simulink model "simulink_MPC"  (R2015a)
settings: Solver=ode45  StartTime=0.0  StopTime=0.015  RelTol=1e-3
values from neighbouring files (symbols this model uses):
  Ts = 1    [initialization_mpc.m]    (also in mpc_model.m = 0.01; mpc_model_working.m = 0.2; mpc_no_linear_model2.m = 0.005)
undefined symbols (not defined in the file or in its folder): alpha, Ao, Bo, Co, Do
settings Model: Creator=estudiante  LastModifiedBy=berme_000

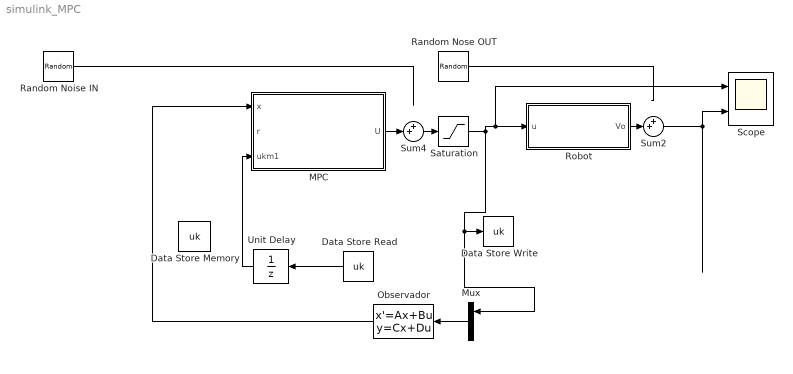
== system simulink_MPC ==
  Data Store Memory : DataStoreMemory  DataStoreName=uk  ReadBeforeWriteMsg=warning  WriteAfterWriteMsg=warning  WriteAfterReadMsg=warning
  Data Store Read : DataStoreRead  DataStoreName=uk
  Data Store Write : DataStoreWrite  DialogController=Simulink.DDGSource  DataStoreName=uk
  MPC : Subsystem
  Mux : Mux  Inputs=2
  Observador : StateSpace  A=Ao  B=Bo  C=Co  D=Do  X0=0
  Random Noise IN : RandomNumber  Variance=.0001  SampleTime=0.0001
  Random Nose OUT : RandomNumber  Variance=0.001  SampleTime=0.0001
  "Robot " : Subsystem
  Saturation : Saturate  UpperLimit=1-alpha  LowerLimit=0.5-alpha
  Scope : Scope  NumInputPorts=2
      settings: TimeRange=0.015  YMin=0.461212~-0.06  YMax=0.50976~0.07
  Sum2 : Sum  Inputs=++|
  Sum4 : Sum  Inputs=++|
  Unit Delay : UnitDelay  SampleTime=-1
  wires:
  Unit Delay/1 -> MPC/3(ukm1)
  Data Store Read/1 -> Unit Delay/1
  Observador/1 -> MPC/1(x)
  Mux/1 -> Observador/1
  Sum2/1 -> Scope/2
  Saturation/1 -> Mux/1, Data Store Write/1, "Robot "/1(u), Scope/1
  MPC/1(U) -> Sum4/2
  Random Noise IN/1 -> ?
  Sum4/1 -> Saturation/1
  "Robot "/1(Vo) -> Sum2/2
  Random Nose OUT/1 -> ?

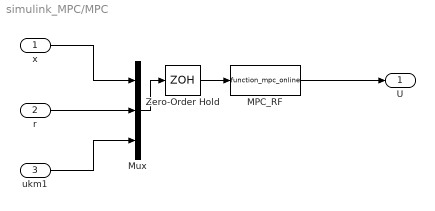
== system simulink_MPC/MPC ==
  x : Inport  PortDimensions=4
  r : Inport  Port=2
  ukm1 : Inport  Port=3
  MPC_RF : MATLABFcn  MATLABFcn=function_mpc_online
  Mux : Mux  Inputs=3
  Zero-Order Hold : ZeroOrderHold  SampleTime=Ts
  U : Outport
  wires:
  x/1 -> Mux/1
  r/1 -> Mux/2
  Mux/1 -> Zero-Order Hold/1
  Zero-Order Hold/1 -> MPC_RF/1
  MPC_RF/1 -> U/1
  ukm1/1 -> Mux/3

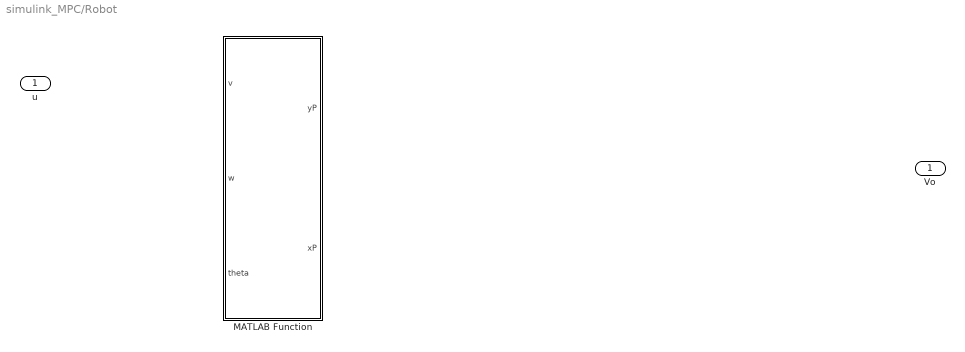
== system simulink_MPC/Robot  ==
  u : Inport
  MATLAB Function : MATLAB Function  TreatAsAtomicUnit=on
  Vo : Outport

== matlab function simulink_MPC/Robot /MATLAB Function ==
  data: v input; w input; yP output; xP output; theta input
function [yP,xP]  = fcn(v,w,theta)
%#codegen
x=v*cos(theta);
y=v*sin(theta);
